simulink library "B_estimatedLib"  (R2023a)
settings: Solver=VariableStepAuto  StartTime=0.0  StopTime=10.0  RelTol=1e-3
settings Model: Creator=afons  LastModifiedBy=afons

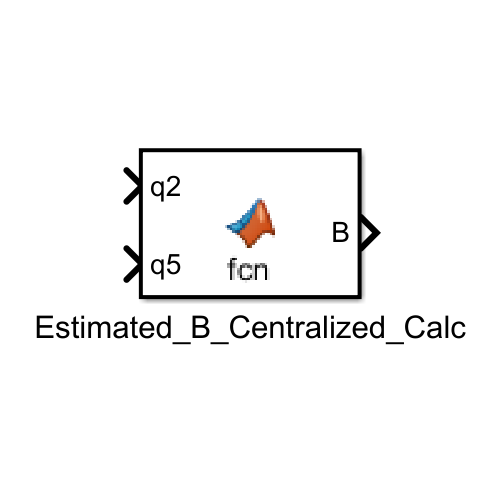
[thumbnail: Simulink's stored preview of the top-level diagram]
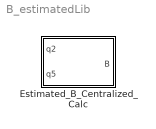
== system B_estimatedLib ==
  Estimated_B_Centralized_Calc : MATLAB Function  TreatAsAtomicUnit=on

== matlab function B_estimatedLib/Estimated_B_Centralized_Calc ==
  data: q2 input; B output; q5 input
function B = Estimated_B_Centralized_Calc(q2,q5)
%#codegen

%    This function was generated by the Symbolic Math Toolbox version 9.3.
%    14-Jun-2023 23:21:33

% q2 = complex(q2);  % if required to enforce complex operations
% q5 = complex(q5);  % if required to enforce complex operations
t2 = q2.*2.0;
t3 = q5.^2;
t4 = pi./9.0;
t5 = pi.*(2.0./9.0);
t6 = pi.*(2.0./1.5e+1);
t7 = pi.*(4.0./1.5e+1);
t8 = pi./4.5e+1;
t12 = pi.*(1.1e+1./4.5e+1);
t9 = cos(t8);
t10 = sin(t8);
t11 = -t8;
t13 = q2+t4;
t14 = q2+t6;
t16 = q2+t12;
t20 = t2+t5;
t26 = t2+t12;
t15 = q2+t11;
t17 = cos(t13);
t18 = sin(t13);
t19 = sin(t14);
t22 = sin(t16);
t23 = cos(t20);
t24 = sin(t20);
t25 = t9.*(3.0./4.0);
t27 = sin(t26);
t21 = sin(t15);
t28 = -t25;
t29 = t18.*pi.*(1.1e+1./6.0);
t30 = t18.*2.402550092724461e+17;
t31 = t19.*1.238489897526886e+18;
t32 = t17.*7.789794370910698e+17;
t33 = q5.*t17.*2.702159776422298e+18;
t34 = -t33;
t35 = t28-2.150524823068501e-1;
t36 = t30+t31+t32+t34;
t37 = t36.*pi.*6.784696261598179e-19;
t38 = -t37;
et1 = q5.*(-8.148409067680494e-1)+t3.*(3.0./2.0)+t9.*6.668416076895004e-2+t10.*2.162102266920123e-1-t17.*1.116396458358791e-2;
et2 = t18.*3.619695120348657e-2-t21.*2.594522720304148e-1-t22.*2.594522720304148e-1;
et3 = t23.*(-1.079715626288445e-1)-t24.*6.099539460032538e-2-t27.*2.162102266920123e-1+cos(q2+t7).*(5.7e+1./1.6e+2);
et4 = cos(t2+t7).*1.85625e-1+cos(q2).*(5.7e+1./1.6e+2)-cos(t6).*5.964178505122713e-2+cos(t7).*1.9890625e-1-cos(t14).*6.539669413511747e-2+cos(t15).*8.002099292274005e-2+cos(t16).*8.002099292274005e-2;
et5 = cos(t26).*6.668416076895004e-2-q5.*t10.*(3.0./4.0)-q5.*t18.*1.255616527394255e-1+q5.*t21.*(9.0./1.0e+1)+q5.*t22.*(9.0./1.0e+1)+q5.*t23.*8.148409067680494e-1+q5.*t24.*2.150524823068501e-1+q5.*t27.*(3.0./4.0)-t3.*t23.*(3.0./2.0);
et6 = pi.^2.*2.054012345679012+5.287192908849745e-1;
mt1 = [et1+et2+et3+et4+et5+et6,t38,t29,t38];
mt2 = [q5.*(-1.629681813536099)+t3.*3.0+t9.*1.333683215379001e-1+t10.*4.324204533840247e-1-q5.*t10.*(3.0./2.0)+6.314923436373623e-1,t35];
mt3 = [t29,t35,3.0];
B = reshape([mt1,mt2,mt3],3,3);
end
